simulink model "spacestate"  (R2018a)
settings: Solver=VariableStepAuto  StartTime=0.0  StopTime=10.0  RelTol=1e-3
settings Model: Creator=gshimabuko  LastModifiedBy=gshimabuko

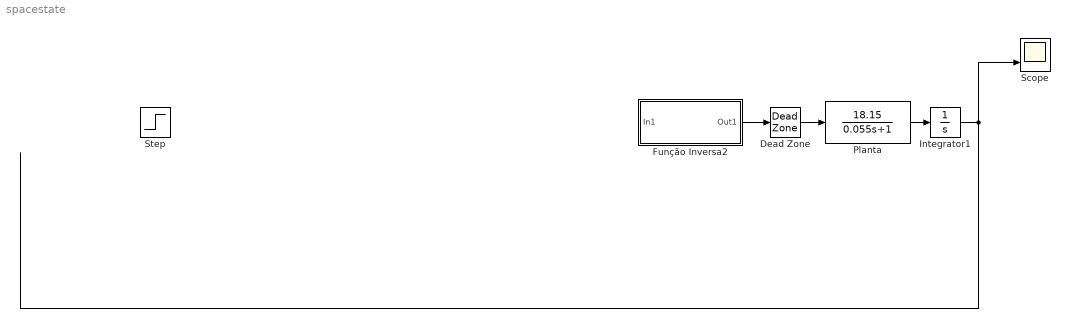
== system spacestate ==
  Dead Zone : DeadZone  LowerValue=-0.7  UpperValue=0.95  SaturateOnIntegerOverflow=on
  Função Inversa2 : Subsystem
  Integrator1 : Integrator
  Planta : TransferFcn  Numerator=[18.15]  Denominator=[0.055 1]
  Scope : Scope  NumInputPorts=2
  Step : Step  SampleTime=0
  wires:
  Planta/1 -> Integrator1/1
  Função Inversa2/1(Out1) -> Dead Zone/1
  Dead Zone/1 -> Planta/1
  ? -> Scope/1
  Integrator1/1 -> Scope/2

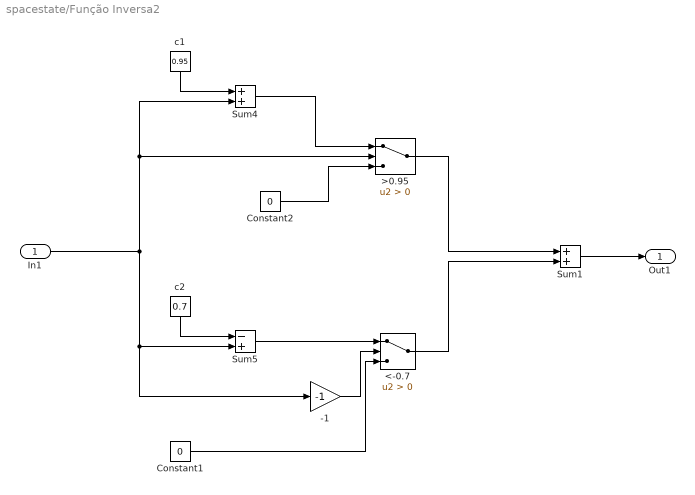
== system spacestate/Função Inversa2 ==
  In1 : Inport
  -1 : Gain  Gain=-1
  "<-0.7 " : Switch  Criteria=u2 > Threshold
  ">0.95 " : Switch  Criteria=u2 > Threshold
  Constant1 : Constant  Value=0
  Constant2 : Constant  Value=0
  Sum1 : Sum
  Sum4 : Sum
  Sum5 : Sum  Inputs=-+
  c1 : Constant  Value=0.95
  c2 : Constant  Value=0.7
  Out1 : Outport
  wires:
  c2/1 -> Sum5/1
  In1/1 -> Sum4/2, ">0.95 "/2, -1/1, Sum5/2
  -1/1 -> "<-0.7 "/2
  Sum5/1 -> "<-0.7 "/1
  Constant1/1 -> "<-0.7 "/3
  "<-0.7 "/1 -> Sum1/2
  ">0.95 "/1 -> Sum1/1
  Sum1/1 -> Out1/1
  c1/1 -> Sum4/1
  Sum4/1 -> ">0.95 "/1
  Constant2/1 -> ">0.95 "/3
